simulink model "SERIAL_TESTE_MCU_CARSIM_4outs"  (R2023b)
settings: Solver=VariableStepAuto  StartTime=0.0  StopTime=12  RelTol=1e-3
libraries: instrumentseriallib x3
settings Model: Creator=Ricardo  LastModifiedBy=Ricardo

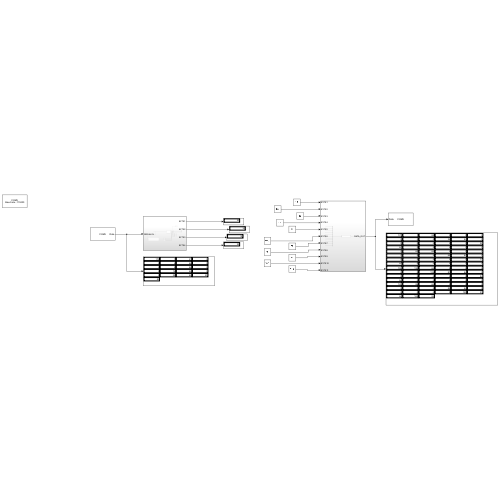
[thumbnail: Simulink's stored preview of the top-level diagram]
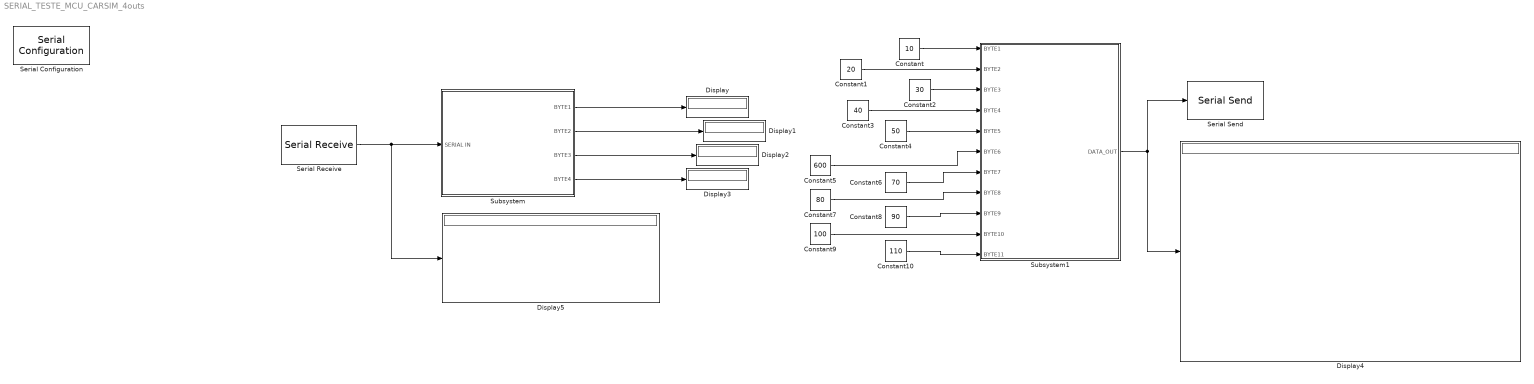
== system SERIAL_TESTE_MCU_CARSIM_4outs ==
  Constant : Constant  Value=10
  Constant1 : Constant  Value=20
  Constant10 : Constant  Value=110
  Constant2 : Constant  Value=30
  Constant3 : Constant  Value=40
  Constant4 : Constant  Value=50
  Constant5 : Constant  Value=600
  Constant6 : Constant  Value=70
  Constant7 : Constant  Value=80
  Constant8 : Constant  Value=90
  Constant9 : Constant  Value=100
  Display{,1..5} (6 alike) : Display
  Serial Configuration : instrumentseriallib/Serial Configuration  Priority=-200000  PortSel=COM5  Port=COM5  ComPort=COM5  BaudRate=115200  DataBits=8  Parity=none  StopBits=1  ByteOrder=little-endian  FlowControl=none  Timeout=10  SimulateUsing=Interpreted execution  BlockInModel=on  aMode=1
      settings: LibrarySourceBlock=embeddedtargetslib/Host Communication/Serial Configuration
  Serial Receive : instrumentseriallib/Serial Receive  Priority=1  PortSel=COM5  Port=COM5  ComPort=COM5  DataType=uint8  SaveDataType=uint8  ToggleHeader=off  Header=[]  ToggleTerminator=on  Terminator=<none>  CustomTerminator=[]  InputFormat=Column major  ToggleDataSize=on  DataSize=21  EnableBlockingMode=on  ActionDataUnavailable=Output last received value  ActionWhenDataUnavailable=Output last received value  CustomValue=0  SampleTime=0.01  SimulateUsing=Interpreted execution  BlockInModel=on  aMode=1
      settings: LibrarySourceBlock=embeddedtargetslib/Host Communication/Serial Receive
  Serial Send : instrumentseriallib/Serial Send  Priority=1  PortSel=COM5  Port=COM5  ComPort=COM5  Header=[]  Terminator=<none>  CustomTerminator=[]  EnableBlockingMode=on  SimulateUsing=Interpreted execution  BlockInModel=on  aMode=1
      settings: LibrarySourceBlock=embeddedtargetslib/Host Communication/Serial Send
  Subsystem : Subsystem
  Subsystem1 : Subsystem
  wires:
  Subsystem/1(BYTE1) -> Display/1
  Subsystem/2(BYTE2) -> Display1/1
  Subsystem/3(BYTE3) -> Display2/1
  Subsystem/4(BYTE4) -> Display3/1
  Constant10/1 -> Subsystem1/11(BYTE11)
  Constant9/1 -> Subsystem1/10(BYTE10)
  Constant6/1 -> Subsystem1/7(BYTE7)
  Constant8/1 -> Subsystem1/9(BYTE9)
  Constant4/1 -> Subsystem1/5(BYTE5)
  Constant7/1 -> Subsystem1/8(BYTE8)
  Constant5/1 -> Subsystem1/6(BYTE6)
  Constant/1 -> Subsystem1/1(BYTE1)
  Constant1/1 -> Subsystem1/2(BYTE2)
  Constant2/1 -> Subsystem1/3(BYTE3)
  Constant3/1 -> Subsystem1/4(BYTE4)
  Subsystem1/1(DATA_OUT) -> Serial Send/1, Display4/1
  Serial Receive/1 -> Display5/1, Subsystem/1(SERIAL IN)

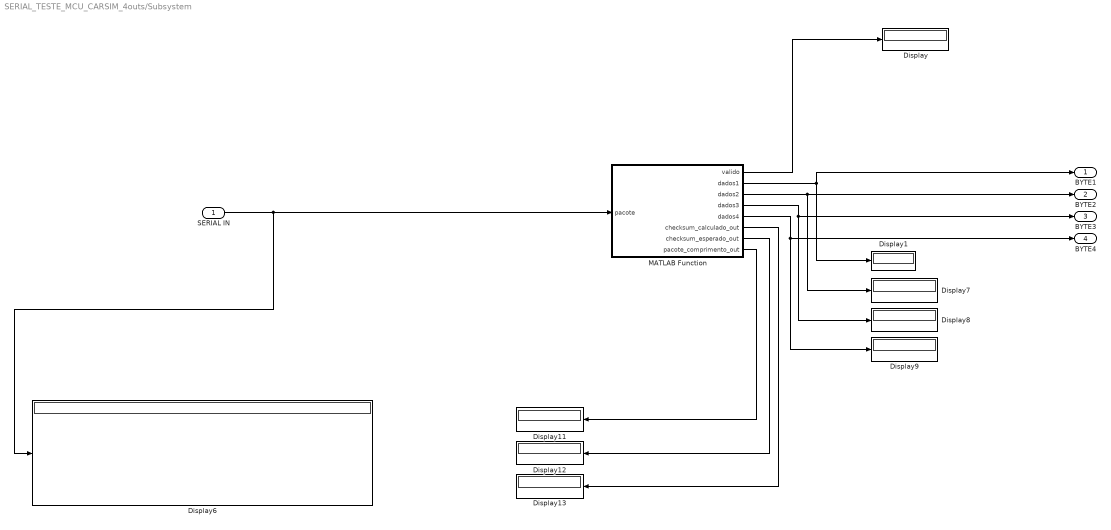
== system SERIAL_TESTE_MCU_CARSIM_4outs/Subsystem ==
  SERIAL IN : Inport
  Display{,1,6..9,11..13} (9 alike) : Display
  MATLAB Function : MATLAB Function  TreatAsAtomicUnit=on
  BYTE1 : Outport
  BYTE2 : Outport  Port=2
  BYTE3 : Outport  Port=3
  BYTE4 : Outport  Port=4
  wires:
  MATLAB Function/4(dados3) -> BYTE3/1, Display8/1
  MATLAB Function/2(dados1) -> BYTE1/1, Display1/1
  MATLAB Function/3(dados2) -> BYTE2/1, Display7/1
  SERIAL IN/1 -> Display6/1, MATLAB Function/1(pacote)
  MATLAB Function/8(pacote_comprimento_out) -> Display11/1
  MATLAB Function/5(dados4) -> BYTE4/1, Display9/1
  MATLAB Function/6(checksum_calculado_out) -> Display13/1
  MATLAB Function/1(valido) -> Display/1
  MATLAB Function/7(checksum_esperado_out) -> Display12/1

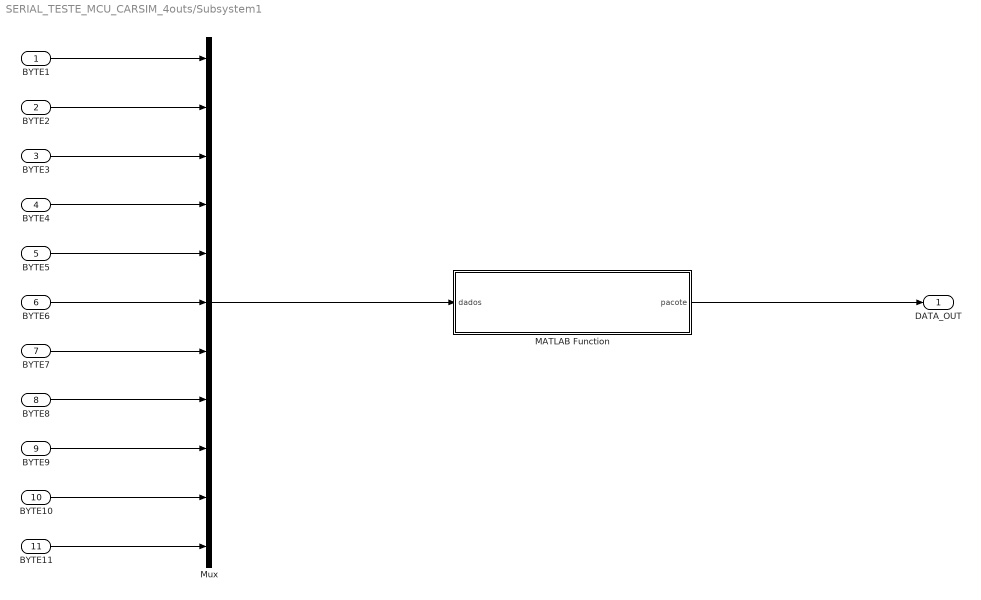
== system SERIAL_TESTE_MCU_CARSIM_4outs/Subsystem1 ==
  BYTE1 : Inport
  BYTE2 : Inport  Port=2
  BYTE3 : Inport  Port=3
  BYTE4 : Inport  Port=4
  BYTE5 : Inport  Port=5
  BYTE6 : Inport  Port=6
  BYTE7 : Inport  Port=7
  BYTE8 : Inport  Port=8
  BYTE9 : Inport  Port=9
  BYTE10 : Inport  Port=10
  BYTE11 : Inport  Port=11
  MATLAB Function : MATLAB Function  TreatAsAtomicUnit=on
  Mux : Mux  Inputs=11
  DATA_OUT : Outport
  wires:
  BYTE7/1 -> Mux/7
  BYTE9/1 -> Mux/9
  BYTE2/1 -> Mux/2
  BYTE1/1 -> Mux/1
  BYTE6/1 -> Mux/6
  BYTE4/1 -> Mux/4
  BYTE10/1 -> Mux/10
  BYTE5/1 -> Mux/5
  BYTE3/1 -> Mux/3
  BYTE11/1 -> Mux/11
  Mux/1 -> MATLAB Function/1(dados)
  BYTE8/1 -> Mux/8
  MATLAB Function/1(pacote) -> DATA_OUT/1

== matlab function SERIAL_TESTE_MCU_CARSIM_4outs/Subsystem1/MATLAB Function ==
  data: dados input; pacote output
function pacote = montar_pacote(dados)
    START_BYTE = uint8(170); % 0xAA
    PACKET_TYPE = uint8(1);  % 0x01 para entrada
    END_BYTE = uint8(85);    % 0x55

    % Garante que dados seja um vetor coluna de 11 elementos
    dados = reshape(dados, [], 1);
    if length(dados) ~= 11
        error('Número incorreto de entradas. Esperado: 11');
    end

    % Converte dados para bytes
    dados_bytes = typecast(dados, 'uint8');
    comprimento = uint8(length(dados_bytes));

    % Verifica se o comprimento dos dados_bytes é 88 (11*8)
    if comprimento ~= 88
        error('Comprimento dos dados bytes incorreto. Esperado: 88');
    end

    % Pré-aloca o pacote com o tamanho correto (93 bytes)
    pacote = zeros(93, 1, 'uint8');

    % Monta o pacote
    pacote(1) = START_BYTE;
    pacote(2) = PACKET_TYPE;
    pacote(3) = comprimento;
    pacote(4:4+length(dados_bytes)-1) = dados_bytes;

    % Calcula e adiciona o checksum
    checksum = calcular_checksum(pacote(2:end-2));
    pacote(end-1) = checksum;
    pacote(end) = END_BYTE;
end

function checksum = calcular_checksum(dados)
    checksum = uint8(0);
    for i = 1:length(dados)
        checksum = bitxor(checksum, uint8(dados(i)));
    end
end

== matlab function SERIAL_TESTE_MCU_CARSIM_4outs/Subsystem/MATLAB Function ==
  data: pacote input; valido output; dados1 output; dados2 output; dados3 output; dados4 output; checksum_calculado_out output; checksum_esperado_out output; pacote_comprimento_out output
function [valido, dados1, dados2, dados3, dados4, checksum_calculado_out, checksum_esperado_out, pacote_comprimento_out] = processar_pacote(pacote)
    % Definir constantes
    START_BYTE = uint8(170); % 0xAA
    END_BYTE = uint8(85); % 0x55
    PACKET_LENGTH = uint8(21); % Novo comprimento esperado do pacote
    DATA_LENGTH = uint8(16); % Novo comprimento dos dados dentro do pacote (4 floats * 4 bytes)

    % Inicializar variáveis de saída
    valido = uint8(0);
    dados1 = single(0);
    dados2 = single(0);
    dados3 = single(0);
    dados4 = single(0);
    checksum_calculado_out = uint8(0);
    checksum_esperado_out = uint8(0);
    pacote_comprimento_out = uint8(0);

    % Verificar comprimento do pacote
    if length(pacote) ~= double(PACKET_LENGTH)
        pacote_comprimento_out = uint8(length(pacote));
        return;
    end

    % Verificar byte de início
    if pacote(1) ~= START_BYTE
        checksum_calculado_out = uint8(pacote(1)); % Use this output to debug the start byte
        return;
    end

    % Verificar byte de fim
    if pacote(end) ~= END_BYTE
        checksum_calculado_out = uint8(pacote(end)); % Use this output to debug the end byte
        return;
    end

    % Extrair os dados e verificar integridade do pacote (checksum)
    dados_bytes = pacote(4:end-2); % Ignorar start byte, tipo e comprimento
    checksum_esperado_out = uint8(pacote(end-1));

    % Calcular checksum usando CheckSum8 XOR
    checksum_calculado = calcular_checksum(pacote(2:end-2));
    checksum_calculado_out = checksum_calculado;

    if checksum_esperado_out ~= checksum_calculado
        return;
    end

    % Verificar comprimento dos dados extraídos
    if length(dados_bytes) ~= double(DATA_LENGTH)
        return;
    end

    % Converter os bytes para valores single e garantir que são escalares
    dados1 = typecast(uint8(dados_bytes(1:4)), 'single');
    dados2 = typecast(uint8(dados_bytes(5:8)), 'single');
    dados3 = typecast(uint8(dados_bytes(9:12)), 'single');
    dados4 = typecast(uint8(dados_bytes(13:16)), 'single');

    % Definir o pacote como válido
    valido = uint8(1);
end

function checksum = calcular_checksum(dados)
    checksum = uint8(0);
    for i = 1:length(dados)
        checksum = bitxor(checksum, uint8(dados(i)));
    end
end
